simulink model "joint_test"  (R2014a)
settings: Solver=ode45  StartTime=0.0  StopTime=10.0  RelTol=1e-3
PostLoadFcn:
  | r1_axis = [0 1 0];
libraries: mblibv1 x21
Description:
  | Copyright 2014 The MathWorks, Inc.
settings Model: Creator=smiller  LastModifiedBy=smiller
settings OptimizationCC: SimCompilerOptimization=off
settings DebuggingCC: MergeDetectMultiDrivingBlocksExec=error  FrameProcessingCompatibilityMsg=error
settings RTWCC: RTWCompilerOptimization=off

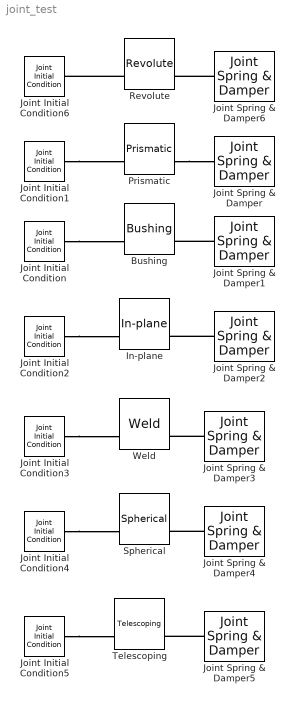
== system joint_test ==
  Bushing : mblibv1/Joints/Bushing  LConnTagsString=__newl0|SA1  RConnTagsString=__newr0|SA1  UpdateFromCAD=off  NumSAPorts=2  CutJoint=off  MarkAsCut=off  Primitives=prismatic_prismatic_prismatic  PrimitiveProps=P1$World$[1 0 0]$prismatic#P2$World$[0 1 0]$prismatic#P3$World$[0 0 1]$prismatic#R1$World$[1 0 0]$revolute#R2$World$[0 1 0]$revolute#R3$World$[0 0 1]$revolute  DialogClass=JointBlock  P1Axis=[1 0 0]  P2Axis=[0 1 0]  P3Axis=[0 0 1]  R1Axis=[1 0 0]  R2Axis=[0 1 0]  R3Axis=[0 0 1]
  In-plane : mblibv1/Joints/In-plane  LConnTagsString=__newl0|SA1  RConnTagsString=__newr0|SA1  UpdateFromCAD=off  NumSAPorts=2  CutJoint=off  MarkAsCut=off  Primitives=prismatic  PrimitiveProps=P1$World$[1 0 0]$prismatic#P2$World$[0 1 0]$prismatic  DialogClass=JointBlock  P1Axis=[1 0 0]  P2Axis=[0 1 0]
  Joint Initial Condition : mblibv1/Sensors &  Actuators/Joint Initial Condition  UpdateFromCAD=off  LeftPortType=blob  RightPortType=blob  PhysicalDomain=mechanical  DialogClass=InitialConditionBlock  InitialConditions=P1$true$1$m$deg$0$m/s$deg/s#P2$true$2$m$deg$0$m/s$deg/s#P3$true$3$m$deg$0$m/s$deg/s#R1$true$4$m$deg$0$m/s$deg/s#R2$true$5$m$deg$0$m/s$deg/s#R3$true$6$m$deg$0$m/s$deg/s#S$false$0$m$deg$0$m/s$deg/s  P1PIC=1  P1VIC=0  P2PIC=2  P2VIC=0  P3PIC=3  P3VIC=0  R1PIC=4  R1VIC=0  R2PIC=5  R2VIC=0  R3PIC=6  R3VIC=0  SPIC=0  SVIC=0
  Joint Initial Condition1 : mblibv1/Sensors &  Actuators/Joint Initial Condition  UpdateFromCAD=off  LeftPortType=blob  RightPortType=blob  PhysicalDomain=mechanical  DialogClass=InitialConditionBlock  InitialConditions=P1$true$h$m$deg$0$m/s$deg/s#P2$false$0$m$deg$0$m/s$deg/s#P3$false$0$m$deg$0$m/s$deg/s#R1$false$0$m$deg$0$m/s$deg/s#R2$false$0$m$deg$0$m/s$deg/s#R3$false$0$m$deg$0$m/s$deg/s#S$false$0$m$deg$0$m/s$deg/s  P1PIC=h  P1VIC=0  P2PIC=0  P2VIC=0  P3PIC=0  P3VIC=0  R1PIC=0  R1VIC=0  R2PIC=0  R2VIC=0  R3PIC=0  R3VIC=0  SPIC=0  SVIC=0
  Joint Initial Condition2 : mblibv1/Sensors &  Actuators/Joint Initial Condition  UpdateFromCAD=off  LeftPortType=blob  RightPortType=blob  PhysicalDomain=mechanical  DialogClass=InitialConditionBlock  InitialConditions=P1$true$1$m$deg$0$m/s$deg/s#P2$true$2$m$deg$0$m/s$deg/s#P3$false$3$m$deg$0$m/s$deg/s#R1$false$4$m$deg$0$m/s$deg/s#R2$false$5$m$deg$0$m/s$deg/s#R3$false$6$m$deg$0$m/s$deg/s#S$false$0$m$deg$0$m/s$deg/s  P1PIC=1  P1VIC=0  P2PIC=2  P2VIC=0  P3PIC=0  P3VIC=0  R1PIC=0  R1VIC=0  R2PIC=0  R2VIC=0  R3PIC=0  R3VIC=0  SPIC=0  SVIC=0
  Joint Initial Condition3 : mblibv1/Sensors &  Actuators/Joint Initial Condition  UpdateFromCAD=off  LeftPortType=blob  RightPortType=blob  PhysicalDomain=mechanical  DialogClass=InitialConditionBlock  InitialConditions=P1$false$1$m$deg$0$m/s$deg/s#P2$false$2$m$deg$0$m/s$deg/s#P3$false$3$m$deg$0$m/s$deg/s#R1$false$4$m$deg$0$m/s$deg/s#R2$false$5$m$deg$0$m/s$deg/s#R3$false$6$m$deg$0$m/s$deg/s#S$false$0$m$deg$0$m/s$deg/s  P1PIC=0  P1VIC=0  P2PIC=0  P2VIC=0  P3PIC=0  P3VIC=0  R1PIC=0  R1VIC=0  R2PIC=0  R2VIC=0  R3PIC=0  R3VIC=0  SPIC=0  SVIC=0
  Joint Initial Condition4 : mblibv1/Sensors &  Actuators/Joint Initial Condition  UpdateFromCAD=off  LeftPortType=blob  RightPortType=blob  PhysicalDomain=mechanical  DialogClass=InitialConditionBlock  InitialConditions=P1$false$1$m$deg$0$m/s$deg/s#P2$false$2$m$deg$0$m/s$deg/s#P3$false$3$m$deg$0$m/s$deg/s#R1$false$4$m$deg$0$m/s$deg/s#R2$false$5$m$deg$0$m/s$deg/s#R3$false$6$m$deg$0$m/s$deg/s#S$false$0$m$deg$0$m/s$deg/s  P1PIC=0  P1VIC=0  P2PIC=0  P2VIC=0  P3PIC=0  P3VIC=0  R1PIC=0  R1VIC=0  R2PIC=0  R2VIC=0  R3PIC=0  R3VIC=0  SPIC=0  SVIC=0
  Joint Initial Condition5 : mblibv1/Sensors &  Actuators/Joint Initial Condition  UpdateFromCAD=off  LeftPortType=blob  RightPortType=blob  PhysicalDomain=mechanical  DialogClass=InitialConditionBlock  InitialConditions=P1$true$1$m$deg$0$m/s$deg/s#P2$false$2$m$deg$0$m/s$deg/s#P3$false$3$m$deg$0$m/s$deg/s#R1$false$4$m$deg$0$m/s$deg/s#R2$false$5$m$deg$0$m/s$deg/s#R3$false$6$m$deg$0$m/s$deg/s#S$false$0$m$deg$0$m/s$deg/s  P1PIC=1  P1VIC=0  P2PIC=0  P2VIC=0  P3PIC=0  P3VIC=0  R1PIC=0  R1VIC=0  R2PIC=0  R2VIC=0  R3PIC=0  R3VIC=0  SPIC=0  SVIC=0
  Joint Initial Condition6 : mblibv1/Sensors &  Actuators/Joint Initial Condition  UpdateFromCAD=off  LeftPortType=blob  RightPortType=blob  PhysicalDomain=mechanical  DialogClass=InitialConditionBlock  InitialConditions=P1$false$h$m$deg$0$m/s$deg/s#P2$false$0$m$deg$0$m/s$deg/s#P3$false$0$m$deg$0$m/s$deg/s#R1$true$1$m$rev$2$m/s$rpm#R2$false$0$m$deg$0$m/s$deg/s#R3$false$0$m$deg$0$m/s$deg/s#S$false$0$m$deg$0$m/s$deg/s  P1PIC=0  P1VIC=0  P2PIC=0  P2VIC=0  P3PIC=0  P3VIC=0  R1PIC=1  R1VIC=2  R2PIC=0  R2VIC=0  R3PIC=0  R3VIC=0  SPIC=0  SVIC=0
  Joint Spring & Damper : mblibv1/Force  Elements/Joint Spring & Damper  UpdateFromCAD=off  DialogClass=JointSpringDamper  JFEParameters=P1$true$1$2$3$cm$in/s$dyn$deg$deg/s$N*m#P2$false$0$0$0$m$m/s$N$deg$deg/s$N*m#P3$false$0$0$0$m$m/s$N$deg$deg/s$N*m#R1$false$0$0$0$m$m/s$N$deg$deg/s$N*m#R2$false$0$0$0$m$m/s$N$deg$deg/s$N*m#R3$false$0$0$0$m$m/s$N$deg$deg/s$N*m#S$false$0$0$0$m$m/s$N$deg$deg/s$N*m
  Joint Spring & Damper1 : mblibv1/Force  Elements/Joint Spring & Damper  UpdateFromCAD=off  DialogClass=JointSpringDamper  JFEParameters=P1$true$1$11$112$m$in/s$N$deg$deg/s$N*m#P2$true$2$22$223$cm$ft/s$lbf$deg$deg/s$N*m#P3$true$3$33$334$mm$mi/s$mN$deg$deg/s$N*m#R1$true$4$44$445$m$m/s$N$rad$rpm$mN*m#R2$true$5$55$556$m$m/s$N$rad$rpm$mN*m#R3$true$6$66$667$m$m/s$N$rad$rpm$mN*m#S$false$0$0$0$m$m/s$N$deg$deg/s$N*m
  Joint Spring & Damper{2..5} (4 alike) : mblibv1/Force  Elements/Joint Spring & Damper  UpdateFromCAD=off  DialogClass=JointSpringDamper  JFEParameters=P1$true$1$11$112$m$in/s$dyn$deg$deg/s$N*m#P2$true$2$22$223$cm$ft/s$lbf$deg$deg/s$N*m#P3$false$3$33$334$mm$mi/s$mN$deg$deg/s$N*m#R1$false$4$44$445$m$m/s$N$rad$rpm$mN*m#R2$false$5$55$556$m$m/s$N$rad$rpm$mN*m#R3$false$6$66$667$m$m/s$N$rad$rpm$mN*m#S$false$0$0$0$m$m/s$N$deg$deg/s$N*m
  Joint Spring & Damper6 : mblibv1/Force  Elements/Joint Spring & Damper  UpdateFromCAD=off  DialogClass=JointSpringDamper  JFEParameters=P1$false$1$2$3$cm$in/s$dyn$deg$deg/s$N*m#P2$false$0$0$0$m$m/s$N$deg$deg/s$N*m#P3$false$0$0$0$m$m/s$N$deg$deg/s$N*m#R1$true$1$2$3$m$m/s$N$rad$rpm$lbf*ft#R2$false$0$0$0$m$m/s$N$deg$deg/s$N*m#R3$false$0$0$0$m$m/s$N$deg$deg/s$N*m#S$false$0$0$0$m$m/s$N$deg$deg/s$N*m
  Prismatic : mblibv1/Joints/Prismatic  LConnTagsString=__newl0|SA1  RConnTagsString=__newr0|SA1  UpdateFromCAD=off  NumSAPorts=2  CutJoint=off  MarkAsCut=off  Primitives=prismatic  PrimitiveProps=P1$Base$[0 0 1]$prismatic  DialogClass=JointBlock  P1Axis=[0 0 1]
  Revolute : mblibv1/Joints/Revolute  LConnTagsString=__newl0|SA1  RConnTagsString=__newr0|SA1  UpdateFromCAD=off  NumSAPorts=2  CutJoint=off  MarkAsCut=off  Primitives=prismatic  PrimitiveProps=R1$World$r1_axis$revolute  DialogClass=JointBlock  R1Axis=r1_axis
  Spherical : mblibv1/Joints/Spherical  LConnTagsString=__newl0|SA1  RConnTagsString=__newr0|SA1  UpdateFromCAD=off  NumSAPorts=2  CutJoint=off  MarkAsCut=off  Primitives=spherical  PrimitiveProps=S$World$[0 0 0]$spherical  DialogClass=JointBlock  SAxis=[0 0 0]
  Telescoping : mblibv1/Joints/Telescoping  LConnTagsString=__newl0|SA1  RConnTagsString=__newr0|SA1  UpdateFromCAD=off  NumSAPorts=2  CutJoint=off  MarkAsCut=off  Primitives=spherical  PrimitiveProps=S$World$[0 0 0]$spherical#P1$World$[1 0 0]$prismatic  DialogClass=JointBlock  SAxis=[0 0 0]  P1Axis=[1 0 0]
  Weld : mblibv1/Joints/Weld  LConnTagsString=__newl0|SA1  RConnTagsString=__newr0|SA1  UpdateFromCAD=off  NumSAPorts=2  CutJoint=off  MarkAsCut=off  Primitives=weld  PrimitiveProps=W$World$[0 0 0]$weld  DialogClass=JointBlock  WAxis=[0 0 0]
  connections:
  Joint Initial Condition/RConn1 -- Bushing/LConn2
  Joint Initial Condition1/RConn1 -- Prismatic/LConn2
  Joint Initial Condition2/RConn1 -- In-plane/LConn2
  Prismatic/RConn2 -- Joint Spring & Damper/LConn1
  Joint Spring & Damper1/LConn1 -- Bushing/RConn2
  Joint Spring & Damper2/LConn1 -- In-plane/RConn2
  Joint Initial Condition3/RConn1 -- Weld/LConn2
  Joint Spring & Damper3/LConn1 -- Weld/RConn2
  Joint Initial Condition4/RConn1 -- Spherical/LConn2
  Joint Spring & Damper4/LConn1 -- Spherical/RConn2
  Joint Spring & Damper5/LConn1 -- Telescoping/RConn2
  Joint Initial Condition5/RConn1 -- Telescoping/LConn2
  Joint Spring & Damper6/LConn1 -- Revolute/RConn2
  Revolute/LConn2 -- Joint Initial Condition6/RConn1
